simulink model "slidingmode_practice_2016"  (R2016b)
settings: Solver=FixedStepAuto  StartTime=0.0  StopTime=200  FixedStep=Ts  RelTol=1e-3  EnableMultiTasking=on
values from neighbouring files (symbols this model uses):
  K1 = 6.1486    [Sliding_mode.m]
  K2 = 6.664    [Sliding_mode.m]
  Ts = 0.02    [Sliding_mode.m]
libraries: simulink x7, raspberrypiBasiclib x6, raspberrypiCommlib x1
settings Model: Creator=hhiastt  LastModifiedBy=hhiastt
settings SolverCC: PositivePriorityOrder=on
settings DataIOCC: ReturnWorkspaceOutputs=on
settings OptimizationCC: EnhancedBackFolding=on  PassReuseOutputArgsAs=Individual arguments  ZeroExternalMemoryAtStartup=off  ZeroInternalMemoryAtStartup=off  MaxStackSize=64
settings DebuggingCC: ParameterTunabilityLossMsg=error
settings HardwareCC: ProdBitPerPointer=32  ProdBitPerSizeT=32  ProdBitPerPtrDiffT=32  ProdLargestAtomicInteger=Long  ProdLargestAtomicFloat=Double  ProdWordSize=32  ProdLongLongMode=on  ProdHWDeviceType=ARM Compatible->ARM Cortex
settings SFSimCC: SimUseLocalCustomCode=on
settings RTWCC: Description=Embedded Coder  SystemTargetFile=ert.tlc  HardwareBoard=Raspberry Pi  TLCOptions="-aInlineSetEventsForThisBaseRateFcn=TLC_FALSE -aSuppressMultiTaskScheduler=TLC_FALSE  -aRateBasedStepFcn=0"  TemplateMakefile=ert_default_tmf  RTWUseLocalCustomCode=on  Toolchain=GNU GCC Raspberry Pi  BuildConfiguration=Faster Runs
settings CodeAppCC: ForceParamTrailComments=on  IgnoreCustomStorageClasses=off  OperatorAnnotations=on  SimulinkDataObjDesc=on  SFDataObjDesc=on  InsertBlockDesc=on
settings ERTTargetCC: MultiwordLength=256  SupportVariableSizeSignals=on

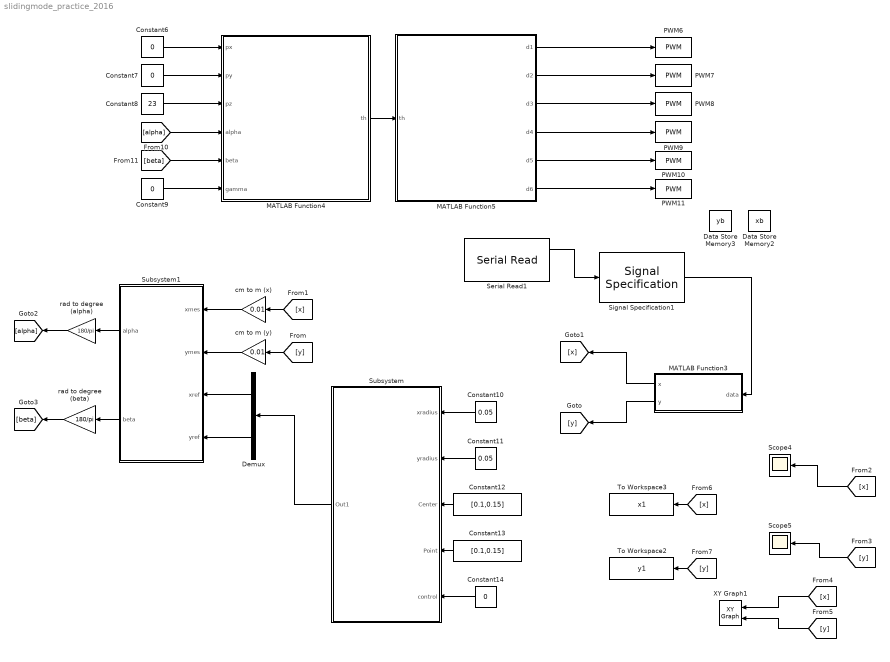
== system slidingmode_practice_2016 ==
  Constant10 : Constant  Value=0.05
  Constant11 : Constant  Value=0.05
  Constant12 : Constant  Value=[0.1,0.15]
  Constant13 : Constant  Value=[0.1,0.15]  VectorParams1D=off
  Constant{6..7,9,14} (4 alike) : Constant  Value=0
  Constant8 : Constant  Value=23
  Data Store Memory2 : DataStoreMemory  DataStoreName=xb  ReadBeforeWriteMsg=warning  WriteAfterWriteMsg=warning  WriteAfterReadMsg=warning  ShowAdditionalParam=off  OutDataTypeStr=double
  Data Store Memory3 : DataStoreMemory  DataStoreName=yb  ReadBeforeWriteMsg=warning  WriteAfterWriteMsg=warning  WriteAfterReadMsg=warning  ShowAdditionalParam=off  OutDataTypeStr=double
  Demux : Demux  Outputs=2
  MATLAB Function3 : MATLAB Function  TreatAsAtomicUnit=on
  MATLAB Function4 : MATLAB Function  TreatAsAtomicUnit=on
  MATLAB Function5 : MATLAB Function  TreatAsAtomicUnit=on
  PWM10 : raspberrypiBasiclib/PWM  board=Pi 3 Model B+  Pin_=27  Frequency=50  blockPlatform=Raspberry Pi
  PWM11 : raspberrypiBasiclib/PWM  board=Pi 3 Model B+  Pin_=22  Frequency=50  blockPlatform=Raspberry Pi
  PWM6 : raspberrypiBasiclib/PWM  board=Pi 3 Model B+  Pin_=12  Frequency=50  blockPlatform=Raspberry Pi
  PWM7 : raspberrypiBasiclib/PWM  board=Pi 3 Model B+  Pin_=20  Frequency=50  blockPlatform=Raspberry Pi
  PWM8 : raspberrypiBasiclib/PWM  board=Pi 3 Model B+  Pin_=16  Frequency=50  blockPlatform=Raspberry Pi
  PWM9 : raspberrypiBasiclib/PWM  board=Pi 3 Model B+  Pin_=17  Frequency=50  blockPlatform=Raspberry Pi
  Scope4 : Scope
  Scope5 : Scope
  Serial Read1 : raspberrypiCommlib/Serial Read  board=Pi 3 Model B+  SCIModule_=/dev/ttyS0  Baudrate_=19200  Parity=None  StopBits_=1  HardwareFlowControl=None  ByteOrder=LittleEndian  DataLength=10  DataType=uint8  OutputStatus=on  SampleTime=Ts  blockPlatform=RaspberryPi
  Signal Specification1 : SignalSpecification  OutDataTypeStr=uint8  Dimensions=10  SampleTime=Ts
  Subsystem : Subsystem
  Subsystem1 : Subsystem
  To Workspace2 : ToWorkspace  VariableName=y1  SampleTime=Ts
      settings: Save2DSignal=2-D array (concatenate along first dimension)
  To Workspace3 : ToWorkspace  VariableName=x1  SampleTime=Ts
      settings: Save2DSignal=2-D array (concatenate along first dimension)
  XY Graph1 : simulink/Sinks/XY Graph  xmin=0  xmax=20  ymin=0  ymax=30  st=Ts
  cm to m (x) : Gain  Gain=0.01
  cm to m (y) : Gain  Gain=0.01
  rad to degree (alpha) : Gain  Gain=180/pi
  rad to degree (beta) : Gain  Gain=180/pi
  wires:
  Subsystem/1(Out1) -> Demux/1
  MATLAB Function5/2(d2) -> PWM7/1
  MATLAB Function4/1(th) -> MATLAB Function5/1(th)
  Constant7/1 -> MATLAB Function4/2(py)
  Constant12/1 -> Subsystem/3(Center)
  [y] -> To Workspace2/1
  MATLAB Function3/1(x) -> [x]
  Constant13/1 -> Subsystem/4(Point)
  Constant10/1 -> Subsystem/1(xradius)
  Demux/1 -> Subsystem1/3(xref)
  [beta] -> MATLAB Function4/5(beta)
  MATLAB Function3/2(y) -> [y]
  cm to m (x)/1 -> Subsystem1/1(xmes)
  [y] -> Scope5/1
  Signal Specification1/1 -> MATLAB Function3/1(data)
  [x] -> Scope4/1
  [y] -> cm to m (y)/1
  MATLAB Function5/4(d4) -> PWM9/1
  MATLAB Function5/6(d6) -> PWM11/1
  [x] -> cm to m (x)/1
  [y] -> XY Graph1/2
  MATLAB Function5/3(d3) -> PWM8/1
  Constant6/1 -> MATLAB Function4/1(px)
  MATLAB Function5/5(d5) -> PWM10/1
  [x] -> XY Graph1/1
  rad to degree (alpha)/1 -> [alpha]
  Constant11/1 -> Subsystem/2(yradius)
  Subsystem1/1(alpha) -> rad to degree (alpha)/1
  MATLAB Function5/1(d1) -> PWM6/1
  Subsystem1/2(beta) -> rad to degree (beta)/1
  [alpha] -> MATLAB Function4/4(alpha)
  Demux/2 -> Subsystem1/4(yref)
  Constant9/1 -> MATLAB Function4/6(gamma)
  cm to m (y)/1 -> Subsystem1/2(ymes)
  [x] -> To Workspace3/1
  Constant8/1 -> MATLAB Function4/3(pz)
  Serial Read1/1 -> Signal Specification1/1
  rad to degree (beta)/1 -> [beta]
  Constant14/1 -> Subsystem/5(control)

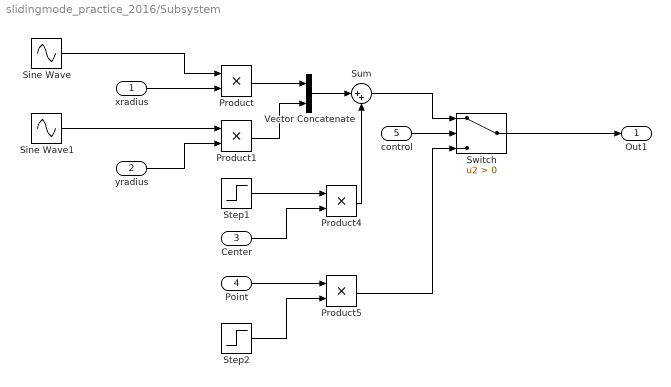
== system slidingmode_practice_2016/Subsystem ==
  xradius : Inport
  yradius : Inport  Port=2
  Center : Inport  Port=3
  Point : Inport  Port=4
  control : Inport  Port=5
  Product{,1,4..5} (4 alike) : Product
  Sine Wave : Sin  Frequency=0.25  SampleTime=Ts
  Sine Wave1 : Sin  Frequency=0.25  Phase=pi/2  SampleTime=Ts
  Step1 : Step  Time=0  SampleTime=Ts
  Step2 : Step  Time=0  SampleTime=Ts
  Sum : Sum  Inputs=|++
  Switch : Switch  Criteria=u2 > Threshold
  Vector Concatenate : Concatenate
  Out1 : Outport
  wires:
  Sine Wave/1 -> Product/1
  Sine Wave1/1 -> Product1/1
  xradius/1 -> Product/2
  yradius/1 -> Product1/2
  Product/1 -> Vector Concatenate/1
  Product1/1 -> Vector Concatenate/2
  Vector Concatenate/1 -> Sum/1
  control/1 -> Switch/2
  Sum/1 -> Switch/1
  Switch/1 -> Out1/1
  Step1/1 -> Product4/1
  Center/1 -> Product4/2
  Product4/1 -> Sum/2
  Point/1 -> Product5/1
  Product5/1 -> Switch/3
  Step2/1 -> Product5/2

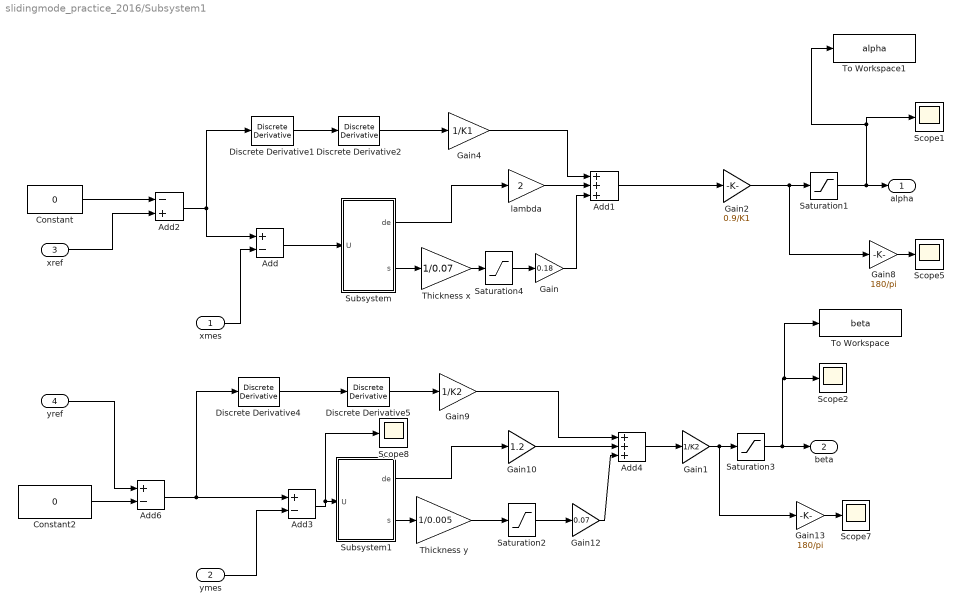
== system slidingmode_practice_2016/Subsystem1 ==
  xmes : Inport
  ymes : Inport  Port=2
  xref : Inport  Port=3
  yref : Inport  Port=4
  Add : Sum  Inputs=+-
  Add1 : Sum  Inputs=+++
  Add2 : Sum  Inputs=-+
  Add3 : Sum  Inputs=+-
  Add4 : Sum  Inputs=+++
  Add6 : Sum  Inputs=+-
  Constant : Constant  Value=0
  Constant2 : Constant  Value=0
  Discrete Derivative{1..2,4..5} (4 alike) : simulink/Discrete/Discrete Derivative  gainval=1.0  ICPrevScaledInput=0.0  OutMin=[]  OutMax=[]  OutDataType=fixdt(1, 16)  OutScaling=2^-10  DoSatur=off
  Gain : Gain  Gain=0.18
  Gain1 : Gain  Gain=1/K2
  Gain10 : Gain  Gain=1.2
  Gain12 : Gain  Gain=0.07
  Gain13 : Gain  Gain=180/pi
  Gain2 : Gain  Gain=0.9/K1
  Gain4 : Gain  Gain=1/K1
  Gain8 : Gain  Gain=180/pi
  Gain9 : Gain  Gain=1/K2
  Saturation1 : Saturate  UpperLimit=5*pi/180  LowerLimit=-5*pi/180  ZeroCross=off
  Saturation2 : Saturate  UpperLimit=1  LowerLimit=-1  ZeroCross=off
  Saturation3 : Saturate  UpperLimit=5*pi/180  LowerLimit=-5*pi/180  ZeroCross=off
  Saturation4 : Saturate  UpperLimit=1  LowerLimit=-1  ZeroCross=off
  Scope{1..2,5,7..8} (5 alike) : Scope
  Subsystem : Subsystem
  Subsystem1 : Subsystem
  Thickness x : Gain  Gain=1/0.07
  Thickness y : Gain  Gain=1/0.005
  To Workspace : ToWorkspace  VariableName=beta  SampleTime=-1
      settings: Save2DSignal=2-D array (concatenate along first dimension)
  To Workspace1 : ToWorkspace  VariableName=alpha  SampleTime=-1
      settings: Save2DSignal=2-D array (concatenate along first dimension)
  lambda : Gain  Gain=2
  alpha : Outport
  beta : Outport  Port=2
  wires:
  Discrete Derivative4/1 -> Discrete Derivative5/1
  Saturation1/1 -> To Workspace1/1, Scope1/1, alpha/1
  Gain8/1 -> Scope5/1
  Add4/1 -> Gain1/1
  Subsystem1/2(s) -> Thickness y/1
  Add3/1 -> Scope8/1, Subsystem1/1(U)
  Discrete Derivative5/1 -> Gain9/1
  Saturation3/1 -> To Workspace/1, Scope2/1, beta/1
  Gain13/1 -> Scope7/1
  Discrete Derivative1/1 -> Discrete Derivative2/1
  Gain/1 -> Add1/3
  Saturation2/1 -> Gain12/1
  Gain12/1 -> Add4/3
  Discrete Derivative2/1 -> Gain4/1
  Gain10/1 -> Add4/2
  lambda/1 -> Add1/2
  Subsystem/2(s) -> Thickness x/1
  Add/1 -> Subsystem/1(U)
  Subsystem/1(de) -> lambda/1
  Gain2/1 -> Gain8/1, Saturation1/1
  Subsystem1/1(de) -> Gain10/1
  Gain1/1 -> Gain13/1, Saturation3/1
  xmes/1 -> Add/2
  Add2/1 -> Add/1, Discrete Derivative1/1
  xref/1 -> Add2/2
  yref/1 -> Add6/1
  ymes/1 -> Add3/2
  Add6/1 -> Discrete Derivative4/1, Add3/1
  Constant/1 -> Add2/1
  Constant2/1 -> Add6/2
  Thickness x/1 -> Saturation4/1
  Thickness y/1 -> Saturation2/1
  Gain4/1 -> Add1/1
  Gain9/1 -> Add4/1
  Saturation4/1 -> Gain/1
  Add1/1 -> Gain2/1

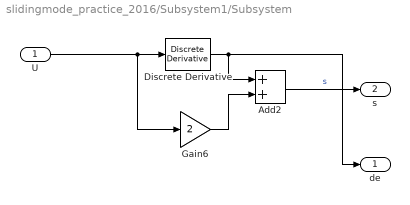
== system slidingmode_practice_2016/Subsystem1/Subsystem ==
  U : Inport
  Add2 : Sum
  Discrete Derivative : simulink/Discrete/Discrete Derivative  gainval=1.0  ICPrevScaledInput=0.0  OutMin=[]  OutMax=[]  OutDataType=fixdt(1, 16)  OutScaling=2^-10  DoSatur=off
  Gain6 : Gain  Gain=2
  de : Outport
  s : Outport  Port=2
  wires:
  Gain6/1 -> Add2/2
  U/1 -> Discrete Derivative/1, Gain6/1
  Discrete Derivative/1 -> de/1, Add2/1
  Add2/1 -> s/1  "s"

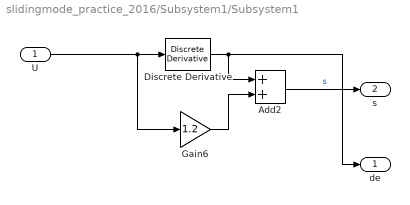
== system slidingmode_practice_2016/Subsystem1/Subsystem1 ==
  U : Inport
  Add2 : Sum
  Discrete Derivative : simulink/Discrete/Discrete Derivative  gainval=1.0  ICPrevScaledInput=0.0  OutMin=[]  OutMax=[]  OutDataType=fixdt(1, 16)  OutScaling=2^-10  DoSatur=off
  Gain6 : Gain  Gain=1.2
  de : Outport
  s : Outport  Port=2
  wires:
  Add2/1 -> s/1  "s"
  Discrete Derivative/1 -> Add2/1, de/1
  U/1 -> Gain6/1, Discrete Derivative/1
  Gain6/1 -> Add2/2

== matlab function slidingmode_practice_2016/MATLAB Function3 ==
  data: data input; x output; y output; xb data_store_memory; yb data_store_memory
function [x,y] = process_data(data)
global xb
global yb
x=0;y=0;xx=0;yy=0;j=0;data1=zeros(1,4);
data2=zeros(1,4);
for i=1:10
    if(data(i) == 255)
        j=i;
    end
end
if(j <= 6 && j>0)
    data1=data(j+1:j+4);
    data2=cast(data1,'like',zeros(1,4));    
    xx=data2(1)*256+data2(2);
    yy=data2(3)*256+data2(4);
    xx=(xx-floor(floor(xx/128)/2)*128)/2;
    yy=(yy-floor(floor(yy/128)/2)*128)/2;
    x=((xx-20)/470)*22.8;
    y=((yy-7)/490)*30.4;
    xb=x;
    yb=y;
else
    x=xb;
    y=yb;
end
end

== matlab function slidingmode_practice_2016/MATLAB Function4 ==
  data: px input double size=1; th output double; py input double size=1; pz input double size=1; alpha input double size=1; beta input double size=1; gamma input double size=1
function th = inv_ken_test(px,py,pz,alpha,beta,gamma)
th=zeros(1,6);
l1=3.2;
l2=25.57;
b=26;
d=20;
b1=30;
d1=6;
RA1=[(1/sqrt(12))*(2*b+d);d/2;0];
RA2=[-(1/sqrt(12))*(b-d);(b+d)/2;0];
RA3=[-(1/sqrt(12))*(b+2*d);b/2;0];
RA4=[-(1/sqrt(12))*(b+2*d);-b/2;0];
RA5=[-(1/sqrt(12))*(b-d);-(b+d)/2;0];
RA6=[(1/sqrt(12))*(2*b+d);-d/2;0];
RA=[RA1 RA2 RA3 RA4 RA5 RA6];

RC1=[(1/sqrt(12))*(b1+2*d1);b1/2;0];
RC2=[(1/sqrt(12))*(b1-d1);(b1+d1)/2;0];
RC3=[-(1/sqrt(12))*(2*b1+d1);d1/2;0];
RC4=[-(1/sqrt(12))*(2*b1+d1);-d1/2;0];
RC5=[(1/sqrt(12))*(b1-d1);-(b1+d1)/2;0];
RC6=[(1/sqrt(12))*(b1+2*d1);-b1/2;0];
RC=[RC1 RC2 RC3 RC4 RC5 RC6];

v=[0 0 0 1];
T_base_A1=[rotz(150)*rotx(90) RA1;v];
T_base_A2=[rotz(-30)*rotx(90) RA2;v];
T_base_A3=[rotz(-90)*rotx(90) RA3;v];
T_base_A4=[rotz(90)*rotx(90) RA4;v];
T_base_A5=[rotz(30)*rotx(90) RA5;v];
T_base_A6=[rotz(-150)*rotx(90) RA6;v];

% Computation
R=[rotz(gamma)*roty(beta)*rotx(alpha);0 0 0];
P=[px;py;pz;1];
T=[R P];
RCE=T*[RC;ones(1,6)];
RAE=[RA;ones(1,6)];
L=zeros(1,6);
for i =1:6
    L(i)=sum((RCE(:,i)-RAE(:,i)).^2)^0.5;
end

RA1C1=T_base_A1^(-1)*(RCE(:,1)-RAE(:,1));
RA2C2=T_base_A2^(-1)*(RCE(:,2)-RAE(:,2));
RA3C3=T_base_A3^(-1)*(RCE(:,3)-RAE(:,3));
RA4C4=T_base_A4^(-1)*(RCE(:,4)-RAE(:,4));
RA5C5=T_base_A5^(-1)*(RCE(:,5)-RAE(:,5));
RA6C6=T_base_A6^(-1)*(RCE(:,6)-RAE(:,6));
RAC=[RA1C1 RA2C2 RA3C3 RA4C4 RA5C5 RA6C6];
P1=zeros(1,6);
G1=zeros(1,6);
for i=1:6
    P1(i)=(L(i)^2+l1^2-l2^2)/(2*l1);
end
for i=1:6
    G1(i)=RAC(1,i)^2+RAC(2,i)^2-(P1(i)^2);
end
delta=1;
for i=1:6
    th(i)=atan2d(P1(i)*RAC(2,i)+RAC(1,i)*delta*sqrt(G1(i)), ...
        abs(P1(i)*RAC(1,i)-RAC(2,i)*delta*sqrt(G1(i))));
end

== matlab function slidingmode_practice_2016/MATLAB Function5 ==
  data: th input double size=6; d1 output double size=1; d2 output; d3 output; d4 output; d5 output; d6 output
function [d1,d2,d3,d4,d5,d6] =    Angle2duty_test(th)
M1=[0,1.14;10,1.23;20,1.29;30,1.38;40,1.45;50,1.53;60,1.61];
p1=polyfit(M1(:,1),M1(:,2),1);
M2=[0,1.67;10,1.76;20,1.83;30,1.91;40,2];
p2=polyfit(M2(:,1),M2(:,2),1);
M3=[0,1.24;10,1.33;20,1.42;30,1.49;40,1.56;50,1.64];
p3=polyfit(M3(:,1),M3(:,2),1);
M4=[0,1.68;10,1.75;20,1.84;30,1.92;37,1.99];
p4=polyfit(M4(:,1),M4(:,2),1);
M5=[0,1.14;10,1.22;20,1.3;30,1.37;40,1.45;50,1.53];
p5=polyfit(M5(:,1),M5(:,2),1);
M6=[0,1.68;10,1.75;20,1.84;26,1.86];
p6=polyfit(M6(:,1),M6(:,2),1);
d=zeros(1,6);
d1=dot(p1,[th(1),1])/20;
d2=dot(p2,[-th(2),1])/20;
d3=dot(p3,[th(3),1])/20;
d4=dot(p4,[-th(4),1])/20;
d5=dot(p5,[th(5),1])/20;
d6=dot(p6,[-th(6),1])/20;
